simulink model "TASK_6_MODEL"  (R2023b)
settings: Solver=VariableStepAuto  StartTime=0.0  StopTime=50
values from neighbouring files (symbols this model uses):
  A = [0,mf*g*h/Jconst,0,-mf*g/Jconst; 1,0,0,0; 0,-g,0,0; 0,0,1,0]    [task6.m]
  B = [1/Jconst;0;0;0]    [task6.m]
  g = 9.81    [task6.m]
  h = 0.1    [task6.m]
  Jconst = mf*h^2+Jb    (= 0.501)    [task6.m]
  kT_pi_d = kpi_d(1:4)-P*C    [task6.m]
  mf = 0.1    [task6.m]
  P = 1/(Cd4*inv(eye(4)-(Ad4-Bd4*kTpi))*Bd4)    [task6.m]
  PI = -kpi(5)    [task6.m]
  PI_d = -kpi_d(5)    [task6.m]
  Ts = 125e-4    (= 0.0125)    [task6.m]
settings Model: Creator=Krish  LastModifiedBy=Krish

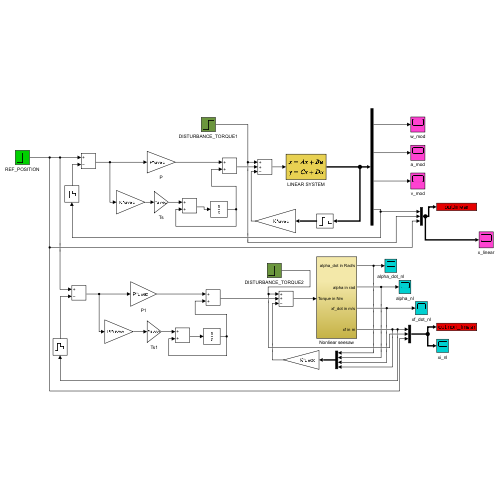
[thumbnail: Simulink's stored preview of the top-level diagram]
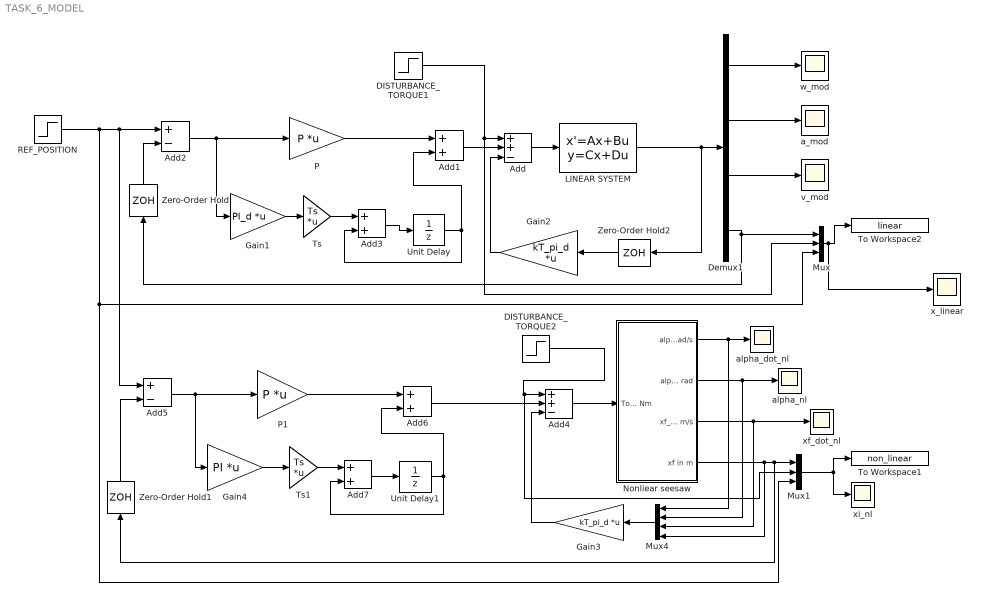
== system TASK_6_MODEL ==
  Add : Sum  Inputs=++-
  Add{1,3,6..7} (4 alike) : Sum
  Add2 : Sum  Inputs=+-
  Add4 : Sum  Inputs=++-
  Add5 : Sum  Inputs=+-
  DISTURBANCE_TORQUE1 : Step  Time=25  After=0.1  SampleTime=0
  DISTURBANCE_TORQUE2 : Step  Time=25  After=0.1  SampleTime=0
  Demux1 : Demux
  Gain1 : Gain  Gain=PI_d  Multiplication=Matrix(K*u) (u vector)
  Gain2 : Gain  Gain=kT_pi_d  Multiplication=Matrix(K*u) (u vector)
  Gain3 : Gain  Gain=kT_pi_d  Multiplication=Matrix(K*u) (u vector)
  Gain4 : Gain  Gain=PI  Multiplication=Matrix(K*u) (u vector)
  LINEAR SYSTEM : StateSpace  A=A  B=B  C=eye(4)  D=[0;0;0;0]  InitialCondition=0
  Mux : Mux  Inputs=3
  Mux1 : Mux  Inputs=3
  Mux4 : Mux
  Nonliear seesaw : Subsystem
  P : Gain  Gain=P  Multiplication=Matrix(K*u) (u vector)
  P1 : Gain  Gain=P  Multiplication=Matrix(K*u) (u vector)
  REF_POSITION : Step  SampleTime=0
  To Workspace1 : ToWorkspace  VariableName=non_linear  SaveFormat=Timeseries  SampleTime=-1
  To Workspace2 : ToWorkspace  VariableName=linear  SaveFormat=Timeseries  SampleTime=-1
  Ts : Gain  Gain=Ts  Multiplication=Matrix(K*u) (u vector)
  Ts1 : Gain  Gain=Ts  Multiplication=Matrix(K*u) (u vector)
  Unit Delay : UnitDelay  InputProcessing=Columns as channels (frame based)  SampleTime=Ts  HasFrameUpgradeWarning=on
  Unit Delay1 : UnitDelay  InputProcessing=Columns as channels (frame based)  SampleTime=Ts  HasFrameUpgradeWarning=on
  Zero-Order Hold : ZeroOrderHold  SampleTime=Ts
  Zero-Order Hold1 : ZeroOrderHold  SampleTime=Ts
  Zero-Order Hold2 : ZeroOrderHold  SampleTime=Ts
  a_mod : Scope
  alpha_dot_nl : Scope
  alpha_nl : Scope
  v_mod : Scope
  w_mod : Scope
  x_linear : Scope
  xf_dot_nl : Scope
  xi_nl : Scope
  wires:
  Add/1 -> LINEAR SYSTEM/1
  REF_POSITION/1 -> Add5/1, Add2/1, Mux1/3, Mux/3
  Add1/1 -> Add/2
  Add2/1 -> Gain1/1, P/1
  Demux1/4 -> Zero-Order Hold/1, Mux/1
  Demux1/3 -> v_mod/1
  Demux1/1 -> w_mod/1
  Gain2/1 -> Add/3
  Demux1/2 -> a_mod/1
  LINEAR SYSTEM/1 -> Zero-Order Hold2/1, Demux1/1
  Unit Delay/1 -> Add3/2, Add1/2
  Add3/1 -> Unit Delay/1
  Zero-Order Hold/1 -> Add2/2
  Mux4/1 -> Gain3/1
  Mux1/1 -> xi_nl/1, To Workspace1/1
  Nonliear seesaw/4(xf in m) -> Mux4/4, Zero-Order Hold1/1, Mux1/1
  Gain3/1 -> Add4/3
  Nonliear seesaw/2(alpha in rad) -> Mux4/2, alpha_nl/1
  Nonliear seesaw/3(xf_dot in m/s) -> Mux4/3, xf_dot_nl/1
  Add4/1 -> Nonliear seesaw/1(Torque in Nm)
  Nonliear seesaw/1(alpha_dot in Rad/s) -> Mux4/1, alpha_dot_nl/1
  Zero-Order Hold1/1 -> Add5/2
  P1/1 -> Add6/1
  Add7/1 -> Unit Delay1/1
  Unit Delay1/1 -> Add6/2, Add7/2
  Gain4/1 -> Ts1/1
  Add5/1 -> Gain4/1, P1/1
  Add6/1 -> Add4/2
  Mux/1 -> To Workspace2/1, x_linear/1
  Zero-Order Hold2/1 -> Gain2/1
  P/1 -> Add1/1
  Gain1/1 -> Ts/1
  Ts/1 -> Add3/1
  DISTURBANCE_TORQUE1/1 -> Mux/2, Add/1
  Ts1/1 -> Add7/1
  DISTURBANCE_TORQUE2/1 -> Mux1/2, Add4/1

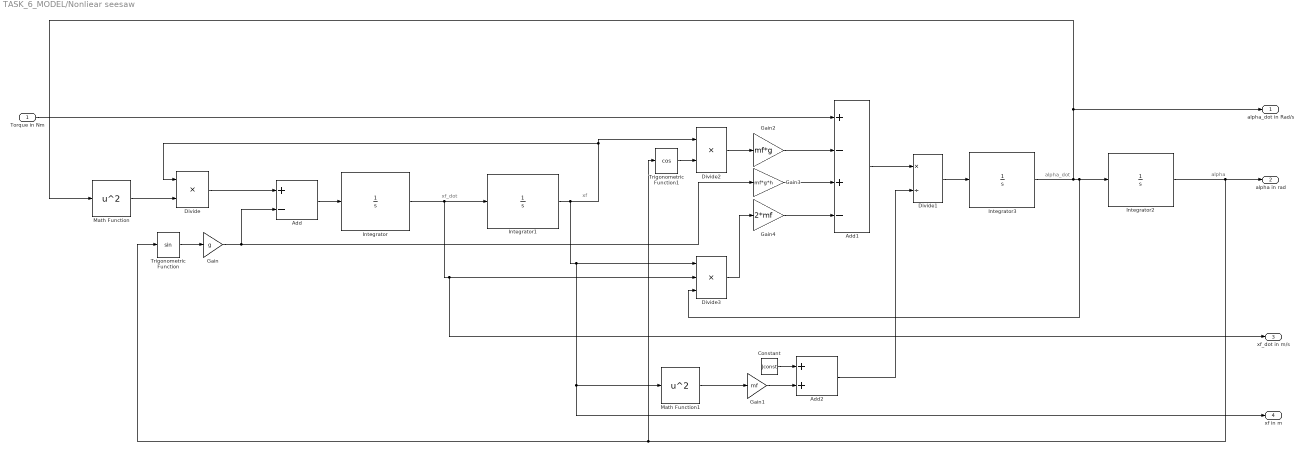
== system TASK_6_MODEL/Nonliear seesaw ==
  note: alpha_dot
  note: xf_dot
  note: xf
  note: alpha
  Torque in Nm : Inport
  Add : Sum  Inputs=+-
  Add1 : Sum  Inputs=+-+-
  Add2 : Sum
  Constant : Constant  Value=Jconst
  Divide : Product  Inputs=**
  Divide1 : Product  Inputs=*/
  Divide2 : Product  Inputs=**
  Divide3 : Product  Inputs=***
  Gain : Gain  Gain=g
  Gain1 : Gain  Gain=mf
  Gain2 : Gain  Gain=mf*g
  Gain3 : Gain  Gain=mf*g*h
  Gain4 : Gain  Gain=2*mf
  Integrator{,1..3} (4 alike) : Integrator
  Math Function : Math  Operator=square
  Math Function1 : Math  Operator=square
  Trigonometric Function : Trigonometry
  Trigonometric Function1 : Trigonometry  Operator=cos
  alpha_dot in Rad/s : Outport
  alpha in rad : Outport  Port=2
  xf_dot in m/s : Outport  Port=3
  xf in m : Outport  Port=4
  wires:
  Gain/1 -> Gain3/1, Add/2
  Integrator2/1 -> Trigonometric Function1/1, Trigonometric Function/1, alpha in rad/1
  Integrator/1 -> xf_dot in m/s/1, Divide3/2, Integrator1/1
  Integrator3/1 -> Integrator2/1, Divide3/3, alpha_dot in Rad/s/1, Math Function/1
  Divide/1 -> Add/1
  Integrator1/1 -> xf in m/1, Math Function1/1, Divide3/1, Divide/1, Divide2/1
  Constant/1 -> Add2/1
  Divide3/1 -> Gain4/1
  Gain2/1 -> Add1/2
  Math Function/1 -> Divide/2
  Add/1 -> Integrator/1
  Gain4/1 -> Add1/4
  Gain1/1 -> Add2/2
  Trigonometric Function/1 -> Gain/1
  Math Function1/1 -> Gain1/1
  Add1/1 -> Divide1/1
  Gain3/1 -> Add1/3
  Divide1/1 -> Integrator3/1
  Add2/1 -> Divide1/2
  Divide2/1 -> Gain2/1
  Trigonometric Function1/1 -> Divide2/2
  Torque in Nm/1 -> Add1/1
